simulink model "model"  (R2024b)
settings: Solver=ode4  StartTime=tspan(1)  StopTime=tspan(2)  FixedStep=h  RelTol=1e-3
values from neighbouring files (symbols this model uses):
  mu = 1    [main.m]
settings Model: Creator=markminerov  LastModifiedBy=markminerov

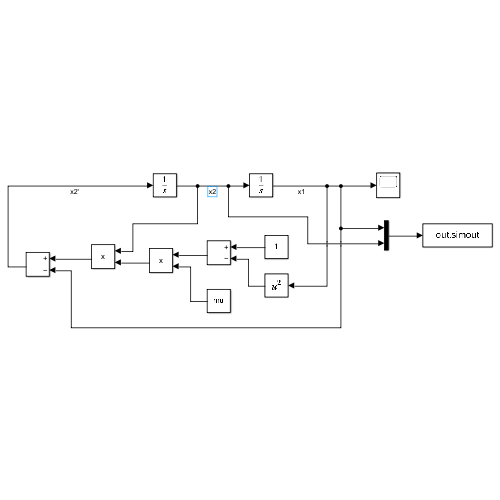
[thumbnail: Simulink's stored preview of the top-level diagram]
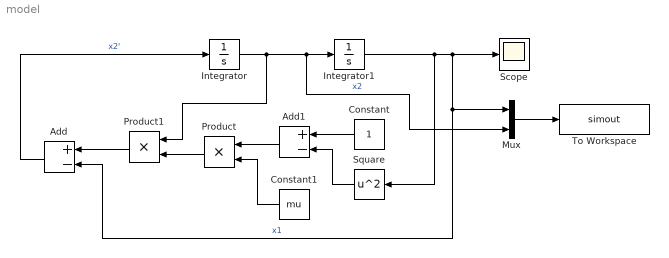
== system model ==
  Add : Sum  Inputs=+-
  Add1 : Sum  Inputs=+-
  Constant : Constant
  Constant1 : Constant  Value=mu
  Integrator : Integrator
  Integrator1 : Integrator  InitialCondition=2
  Mux : Mux  Inputs=2
  Product : Product
  Product1 : Product
  Scope : Scope
  Square : Math  Operator=square
  To Workspace : ToWorkspace  VariableName=simout  SaveFormat=Timeseries  SampleTime=-1
  wires:
  Integrator1/1 -> Add/2, Mux/1, Scope/1, Square/1  "x1"
  Integrator/1 -> Product1/1, Mux/2, Integrator1/1  "x2"
  Add/1 -> Integrator/1  "x2'"
  Constant/1 -> Add1/1
  Square/1 -> Add1/2
  Add1/1 -> Product/1
  Constant1/1 -> Product/2
  Product/1 -> Product1/2
  Product1/1 -> Add/1
  Mux/1 -> To Workspace/1
